simulink library "vehicle_sim_lib"  (R2025b)
settings: Solver=VariableStepAuto  StartTime=0.0  StopTime=10.0  RelTol=1e-3
libraries: controls x1, vehdynlibsteering x1, tire x1, autolibshared x1, battery x1, powertrain x1
settings Model: Creator=jessi  LastModifiedBy=Aditya

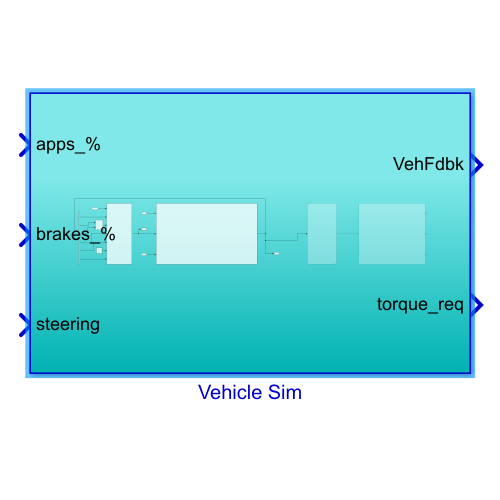
[thumbnail: Simulink's stored preview of the top-level diagram]
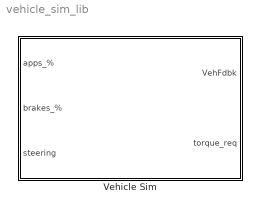
== system vehicle_sim_lib ==
  Vehicle Sim : Subsystem

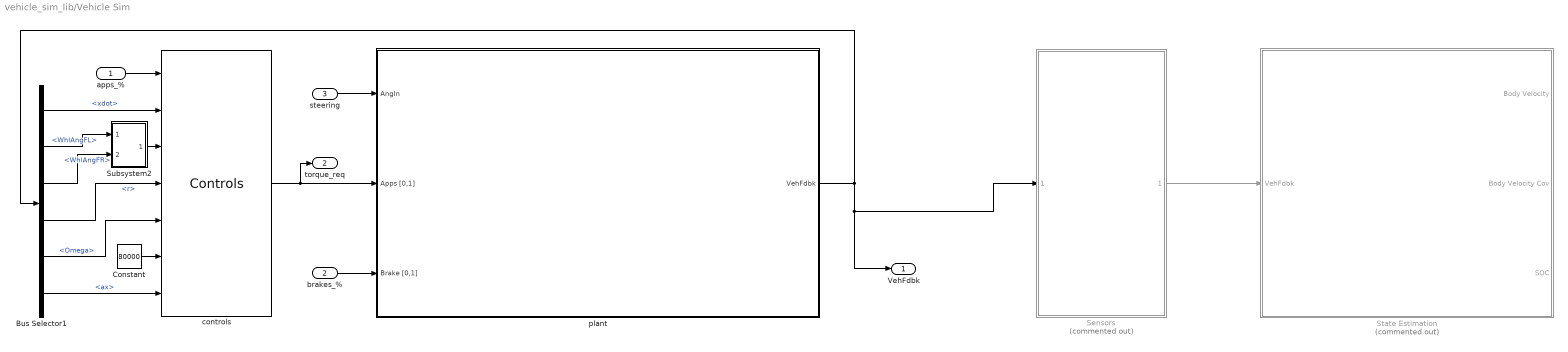
== system vehicle_sim_lib/Vehicle Sim ==
  apps_% : Inport  Unit=%
  brakes_% : Inport  Port=2  PortDimensions=1
  steering : Inport  Port=3
  Bus Selector1 : BusSelector  OutputSignals=BdyFrm.Cg.Vel.xdot,BdyFrm.FrntAxl.Steer.WhlAngFL,BdyFrm.FrntAxl.Steer.WhlAngFR,BdyFrm.Cg.AngVel.r,Wheels.Omega,BdyFrm.Cg.Acc.ax
  Constant : Constant  Value=80000
  Sensors : Subsystem  Commented=on  ReferencedSubsystem=sensor
  State Estimation : Subsystem  Commented=on
  Subsystem2 : Subsystem
  controls : controls/Controls  SystemSampleTime=-1  VariantActivationTime=update diagram  EmptyChoice=off  PassThrough=off  PassThroughVariantControl=(default)  EmptyChoiceVariantControl=(default)  AllowFlexibleInterface=on  Latency=0  AutoFrameSizeCalculation=off
  plant : Subsystem
  VehFdbk : Outport
  torque_req : Outport  Port=2
  wires:
  apps_%/1 -> controls/1
  Bus Selector1/1 -> controls/2  "<xdot>"
  Bus Selector1/4 -> controls/4  "<r>"
  Subsystem2/1(Out1) -> controls/3
  Bus Selector1/2 -> Subsystem2/1(ang1)  "<WhlAngFL>"
  Bus Selector1/3 -> Subsystem2/2(ang2)  "<WhlAngFR>"
  steering/1 -> plant/1(AngIn)
  controls/1 -> torque_req/1, plant/2(Apps [0,1])
  brakes_%/1 -> plant/3(Brake [0,1])
  plant/1(VehFdbk) -> Bus Selector1/1, VehFdbk/1, Sensors/1
  Sensors/1 -> State Estimation/1(VehFdbk)
  Bus Selector1/5 -> controls/5  "<Omega>"
  Bus Selector1/6 -> controls/7  "<ax>"
  Constant/1 -> controls/6

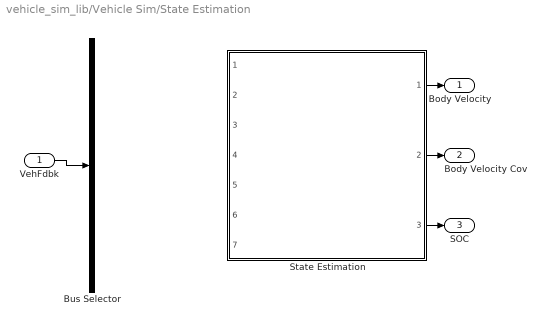
== system vehicle_sim_lib/Vehicle Sim/State Estimation ==
  VehFdbk : Inport
  Bus Selector : BusSelector  OutputSignals=BdyFrm.Cg.Acc.ax,BdyFrm.Cg.Acc.ay,BdyFrm.Cg.AngVel.r
  State Estimation : Subsystem  ReferencedSubsystem=state_estimation
  Body Velocity : Outport
  Body Velocity Cov : Outport  Port=2
  SOC : Outport  Port=3
  wires:
  State Estimation/3 -> SOC/1
  State Estimation/2 -> Body Velocity Cov/1
  State Estimation/1 -> Body Velocity/1
  VehFdbk/1 -> Bus Selector/1

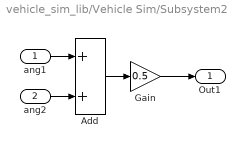
== system vehicle_sim_lib/Vehicle Sim/Subsystem2 ==
  ang1 : Inport
  ang2 : Inport  Port=2
  Add : Sum
  Gain : Gain  Gain=0.5
  Out1 : Outport
  wires:
  ang2/1 -> Add/2
  ang1/1 -> Add/1
  Add/1 -> Gain/1
  Gain/1 -> Out1/1

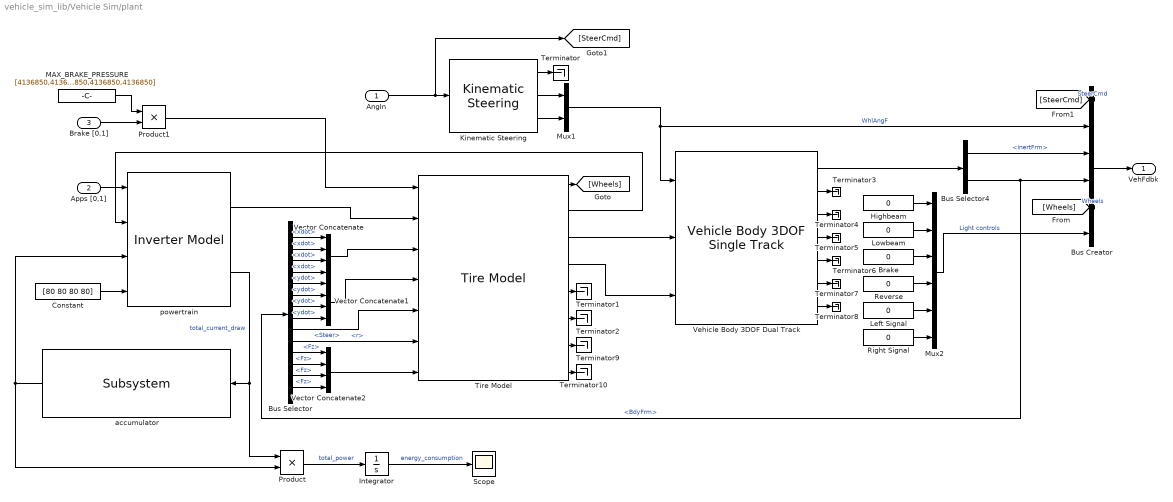
== system vehicle_sim_lib/Vehicle Sim/plant ==
  AngIn : Inport
  Apps [0,1] : Inport  Port=2
  Brake [0,1] : Inport  Port=3
  Brake : Constant  Value=0
  Bus Creator : BusCreator  Inputs=6
  Bus Selector : BusSelector  OutputSignals=FrntAxl.Lft.Vel.xdot,FrntAxl.Rght.Vel.xdot,RearAxl.Lft.Vel.xdot,RearAxl.Rght.Vel.xdot,FrntAxl.Lft.Vel.ydot,FrntAxl.Rght.Vel.ydot,RearAxl.Lft.Vel.ydot,RearAxl.Rght.Vel.ydot,FrntAxl.Steer,Cg.AngVel.r,Forces.Tires.FrntTires.Lft.Fz,Forces.Tires.FrntTires.Rght.Fz,Forces.Tires.RearTires.Lft.Fz,Forces.Tires.RearTires.Rght.Fz
  Bus Selector4 : BusSelector  OutputSignals=InertFrm,BdyFrm
  Constant : Constant  Value=[80 80 80 80]
  Highbeam : Constant  Value=0
  Integrator : Integrator
  Kinematic Steering : vehdynlibsteering/Kinematic Steering  StrgType=Ackerman  StrgRatioType=Constant  Loc=Front  NrmlFctr=1  TrckWdth=1.1  WhlBase=1.550  Db=0  StrgRng=3*pi  StrgAngBpts="[-6.2832   -5.0265   -3.7699   -2.5133   -1.2566         0    1.2566    2.5133    3.7699    5.0265    6.2832]"  StrgRatioTbl=|  StrgRatio=10  PctAckIn=off  PctAck=100  PctAckTbl=ones(1,11)*100  StrgArmLngth=0.1  RckCsLngth=0.5  TieRodLngth=0.248  D=0.2  PnnRadius=0.00085818  PnnRadiusTbl="[0.0055    0.0055    0.0056    0.0057    0.0058    0.0057    0.0057    0.0057    0.0056    0.0055    0.0055]"  RodLngth=0.1  ParaArmLngth=0.9  aMode=2
      | [13.5000   13.3750   13.2500   13.1250   13.0000   13.0000   13.0000   13.1250   13.2500   13.3750   13.5000
      | ]
  Left Signal : Constant  Value=0
  Lowbeam : Constant  Value=0
  MAX_BRAKE_PRESSURE : Constant  Value=[4136850,4136850,4136850,4136850]
  Mux1 : Mux  Inputs=2
  Mux2 : Mux  Inputs=6
  Product : Product
  Product1 : Product
  Reverse : Constant  Value=0
  Right Signal : Constant  Value=0
  Scope : Scope
      settings: ActiveDisplayYMinimum=-1  ActiveDisplayYMaximum=1
  Terminator{,1..10} (11 alike) : Terminator
  Tire Model : tire/Tire Model  SystemSampleTime=-1  VariantActivationTime=update diagram  EmptyChoice=off  PassThrough=off  PassThroughVariantControl=(default)  EmptyChoiceVariantControl=(default)  AllowFlexibleInterface=on  Latency=0  AutoFrameSizeCalculation=off
  Vector Concatenate : Concatenate  NumInputs=4
  Vector Concatenate1 : Concatenate  NumInputs=4
  Vector Concatenate2 : Concatenate  NumInputs=4
  Vehicle Body 3DOF Dual Track : autolibshared/Vehicle Body 3DOF Single Track  trackMode=Dual  inputMode=External forces  frontSteerMode=on  rearSteerMode=off  windMode=off  muMode=off  extFMode=off  extMMode=off  htchFMode=off  htchMMode=off  extXo=off  extpsio=off  extxdoto=off  extro=off  extYo=off  extTamb=off  extydoto=off  aMode=2  NF=2  NR=2  m=300  a=0.837  b=0.713  h=0.30  dh=1  hh=0.2  X_o=0  xdot_o=0  CalphaMode=off  sigmaMode=on  d=0  hl=0  w=[1.1,1.1]  Cy_f=12e3  Cy_r=11e3  sigma_f=.1  sigma_r=.1  alpha_f_brk=[-.1 .1]  Cy_f_data=[-9e3 9e3]  alpha_r_brk=[-.1 .1]  Cy_r_data=[-9e3 9e3]  Y_o=0  ydot_o=0  Izz=4000  psi_o=0  r_o=0  Af=2  Cd=.3  Cl=.1  Cpm=.1  beta_w=[0 0.01:0.01:0.3]  Cs=[0:0.03:0.9]  Cym=[0 1e-6:0.01:0.3]  Pabs=101325  Tair=303  g=9.81  mu=1  xdot_tol=.01  Fznom=1961  Fxtire_sat=7e4  Fytire_sat=7e4  longOff=0  latOff=0  vertOff=0  wrapAng=off
      settings: LibrarySourceBlock=vehdynlibeom/Vehicle Body 3DOF Dual Track
  accumulator : battery/Subsystem  SystemSampleTime=-1  VariantActivationTime=update diagram  EmptyChoice=off  PassThrough=off  PassThroughVariantControl=(default)  EmptyChoiceVariantControl=(default)  AllowFlexibleInterface=on  Latency=0  AutoFrameSizeCalculation=off
  powertrain : powertrain/Inverter Model  SystemSampleTime=-1  VariantActivationTime=update diagram  EmptyChoice=off  PassThrough=off  PassThroughVariantControl=(default)  EmptyChoiceVariantControl=(default)  AllowFlexibleInterface=on  Latency=0  AutoFrameSizeCalculation=off
  VehFdbk : Outport
  wires:
  Vector Concatenate2/1 -> Tire Model/7
  Lowbeam/1 -> Mux2/2
  Vector Concatenate/1 -> Tire Model/3
  powertrain/1 -> Tire Model/2
  Tire Model/3 -> Vehicle Body 3DOF Dual Track/2
  Bus Selector/14 -> Vector Concatenate2/4  "<Fz>"
  Kinematic Steering/3 -> Mux1/2
  Vector Concatenate1/1 -> Tire Model/4
  [Wheels] -> Bus Creator/5  "Wheels"
  powertrain/2 -> Product/1, accumulator/1  "total_current_draw"
  Vehicle Body 3DOF Dual Track/2 -> Terminator3/1
  Bus Selector/9 -> Tire Model/5  "<Steer>"
  Bus Selector/10 -> Tire Model/6  "<r>"
  MAX_BRAKE_PRESSURE/1 -> Product1/1
  Bus Selector/2 -> Vector Concatenate/2  "<xdot>"
  Mux2/1 -> Bus Creator/6  "Light controls"
  [SteerCmd] -> Bus Creator/1  "SteerCmd"
  Tire Model/1 -> [Wheels]
  Integrator/1 -> Scope/1  "energy_consumption"
  Vehicle Body 3DOF Dual Track/1 -> Bus Selector4/1
  Bus Selector4/1 -> Bus Creator/3  "<InertFrm>"
  Tire Model/2 -> powertrain/2
  Apps [0,1]/1 -> powertrain/1
  Highbeam/1 -> Mux2/1
  Bus Selector/12 -> Vector Concatenate2/2  "<Fz>"
  Tire Model/4 -> Vehicle Body 3DOF Dual Track/3
  Brake/1 -> Mux2/3
  Kinematic Steering/2 -> Mux1/1
  Vehicle Body 3DOF Dual Track/7 -> Terminator8/1
  Bus Creator/1 -> VehFdbk/1
  Right Signal/1 -> Mux2/6
  AngIn/1 -> [SteerCmd], Kinematic Steering/1
  Product1/1 -> Tire Model/1
  accumulator/1 -> Product/2, powertrain/3
  Bus Selector/8 -> Vector Concatenate1/4  "<ydot>"
  Vehicle Body 3DOF Dual Track/4 -> Terminator5/1
  Bus Selector/4 -> Vector Concatenate/4  "<xdot>"
  Kinematic Steering/1 -> Terminator/1
  Bus Selector/6 -> Vector Concatenate1/2  "<ydot>"
  Vehicle Body 3DOF Dual Track/3 -> Terminator4/1
  Bus Selector/1 -> Vector Concatenate/1  "<xdot>"
  Product/1 -> Integrator/1  "total_power"
  Vehicle Body 3DOF Dual Track/6 -> Terminator7/1
  Bus Selector/5 -> Vector Concatenate1/1  "<ydot>"
  Bus Selector/11 -> Vector Concatenate2/1  "<Fz>"
  Bus Selector/13 -> Vector Concatenate2/3  "<Fz>"
  Bus Selector/7 -> Vector Concatenate1/3  "<ydot>"
  Bus Selector4/2 -> Bus Creator/4, Bus Selector/1  "<BdyFrm>"
  Vehicle Body 3DOF Dual Track/5 -> Terminator6/1
  Reverse/1 -> Mux2/4
  Left Signal/1 -> Mux2/5
  Mux1/1 -> Bus Creator/2, Vehicle Body 3DOF Dual Track/1  "WhlAngF"
  Constant/1 -> powertrain/4
  Bus Selector/3 -> Vector Concatenate/3  "<xdot>"
  Brake [0,1]/1 -> Product1/2
  Tire Model/5 -> Terminator1/1
  Tire Model/6 -> Terminator2/1
  Tire Model/7 -> Terminator9/1
  Tire Model/8 -> Terminator10/1
